simulink model "parte_2"  (R2017b)
settings: Solver=VariableStepAuto  StartTime=0.0  StopTime=10.0  RelTol=1e-3
libraries: simulink x2
settings Model: Creator=Familia Hernández  LastModifiedBy=Familia Hernández

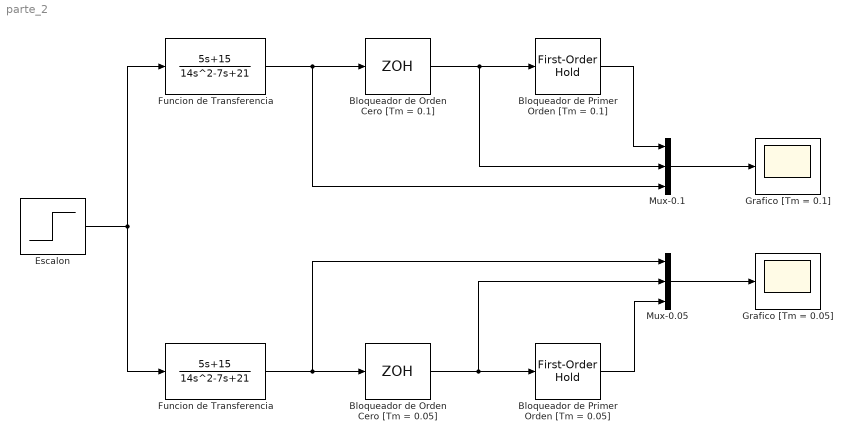
== system parte_2 ==
  Bloqueador de Orden Cero [Tm = 0.05] : ZeroOrderHold  SampleTime=0.05
  Bloqueador de Orden Cero [Tm = 0.1] : ZeroOrderHold  SampleTime=0.1
  Bloqueador de Primer Orden [Tm = 0.05] : simulink/Discrete/First-Order Hold  DisableCoverage=on  Ts=0.05
      settings: SourceProductName=Simulink  SourceProductBaseCode=SL
  Bloqueador de Primer Orden [Tm = 0.1] : simulink/Discrete/First-Order Hold  DisableCoverage=on  Ts=0.1
      settings: SourceProductName=Simulink  SourceProductBaseCode=SL
  Escalon : Step  SampleTime=0
  Funcion de Transferencia : TransferFcn  Numerator=[0 5 15]  Denominator=[14 -7 21]
  "Funcion de Transferencia " : TransferFcn  Numerator=[0 5 15]  Denominator=[14 -7 21]
  Grafico [Tm = 0.05] : Scope
  Grafico [Tm = 0.1] : Scope
  Mux-0.05 : Mux  Inputs=3
  Mux-0.1 : Mux  Inputs=3
  wires:
  Escalon/1 -> "Funcion de Transferencia "/1, Funcion de Transferencia/1
  Mux-0.1/1 -> Grafico [Tm = 0.1]/1
  Funcion de Transferencia/1 -> Mux-0.1/3, Bloqueador de Orden Cero [Tm = 0.1]/1
  Bloqueador de Orden Cero [Tm = 0.1]/1 -> Mux-0.1/2, Bloqueador de Primer Orden [Tm = 0.1]/1
  Bloqueador de Primer Orden [Tm = 0.1]/1 -> Mux-0.1/1
  Bloqueador de Orden Cero [Tm = 0.05]/1 -> Mux-0.05/2, Bloqueador de Primer Orden [Tm = 0.05]/1
  Mux-0.05/1 -> Grafico [Tm = 0.05]/1
  "Funcion de Transferencia "/1 -> Mux-0.05/1, Bloqueador de Orden Cero [Tm = 0.05]/1
  Bloqueador de Primer Orden [Tm = 0.05]/1 -> Mux-0.05/3
